simulink model "FirmwareArchitecture"  (R2024a)
settings: Solver=FixedStepDiscrete  StartTime=0.0  StopTime=10.0  RelTol=1e-3
settings Model: DataDictionary=data_definitions.sldd  Creator=pedro  LastModifiedBy=pedro

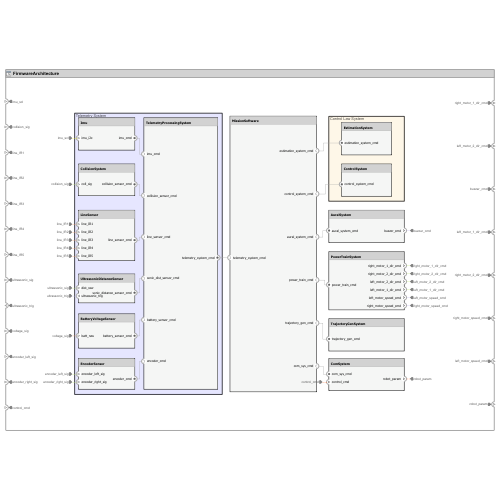
[thumbnail: Simulink's stored preview of the top-level diagram]
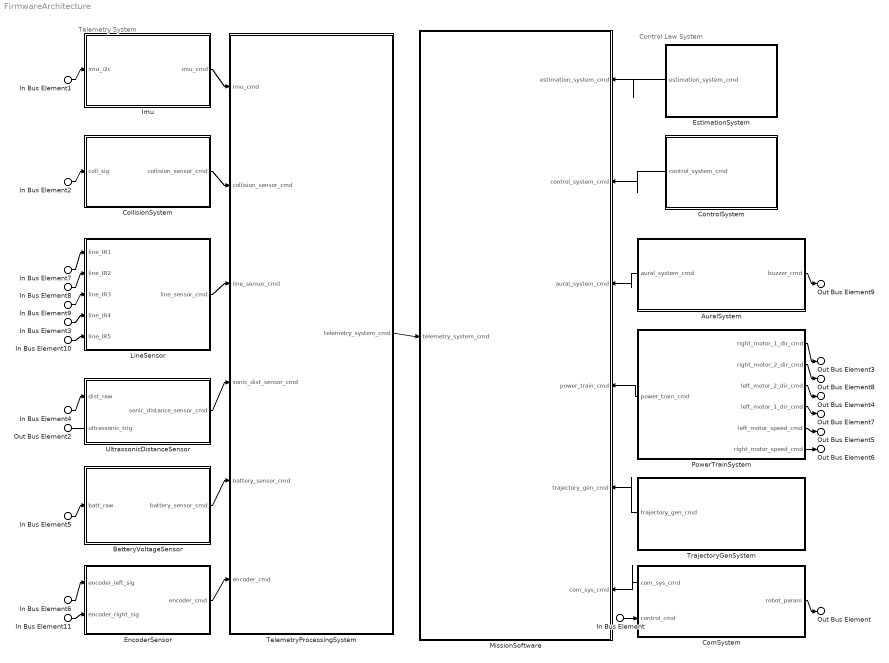
== system FirmwareArchitecture ==
  note: Control Law System
  note: Telemetry System
  In Bus Element1 : Inport  PortName=imu_scl
  In Bus Element2 : Inport  Port=2  PortName=collision_sig
  In Bus Element7 : Inport  Port=3  PortName=line_IR1
  In Bus Element8 : Inport  Port=4  PortName=line_IR2
  In Bus Element9 : Inport  Port=5  PortName=line_IR3
  In Bus Element3 : Inport  Port=6  PortName=line_IR4
  In Bus Element10 : Inport  Port=7  PortName=line_IR5
  In Bus Element4 : Inport  Port=8  PortName=ultrassonic_sig
  In Bus Element5 : Inport  Port=9  PortName=voltage_sig
  In Bus Element6 : Inport  Port=10  PortName=encoder_left_sig
  In Bus Element11 : Inport  Port=11  PortName=encoder_right_sig
  In Bus Element : Inport  Port=12  PortName=control_cmd
  AuralSystem : Subsystem
      settings: PortSchema="{\"entries\":[{\"content\":{\"headerSize\":26,\"margin\":15,\"minimumSpacing\":25,\"sides\":[{\"content\":{\"connectorIds\":[\"Out2\"]},\"type\":\"ConnectorPlacement.EquallySpacedRectSide\",\"uuid\":\"4d6c5e10-6186-41fb-b2bf-ba98d7aba04e\"},{\"content\":{\"connectorIds\":[\"Out1\"],\"side\":\"RIGHT\"},\"type\":\"ConnectorPlacement.EquallySpacedRectSide\",\"uuid\":\"376cbcb5-ae00-4ee4-b51a-d7e41488d4d0\"},{\"content\":{\"side\":\"TOP\"},\"type\":\"ConnectorPlacement.EquallySpacedRectSide\",\"uuid\":\"7d78b6f2-ded8-4819-b676-701e54dd8720\"}]},\"type\":\"ConnectorPlacement.EquallySpacedConnector\",\"uuid\":\"61036d85-7ed2-4698-95df-f6a26735d595\"}],\"packageUris\":[\"http://schema.mathworks.com/mf0/Connector/R2020b\"],\"version\":\"1.0\"}"
  BatteryVoltageSensor : Subsystem
      settings: PortSchema="{\"entries\":[{\"content\":{\"headerSize\":26,\"margin\":15,\"minimumSpacing\":25,\"sides\":[{\"content\":{\"connectorIds\":[\"In1\"]},\"type\":\"ConnectorPlacement.EquallySpacedRectSide\",\"uuid\":\"4d6c5e10-6186-41fb-b2bf-ba98d7aba04e\"},{\"content\":{\"connectorIds\":[\"Out1\"],\"side\":\"RIGHT\"},\"type\":\"ConnectorPlacement.EquallySpacedRectSide\",\"uuid\":\"376cbcb5-ae00-4ee4-b51a-d7e41488d4d0\"},{\"content\":{\"side\":\"TOP\"},\"type\":\"ConnectorPlacement.EquallySpacedRectSide\",\"uuid\":\"7d78b6f2-ded8-4819-b676-701e54dd8720\"}]},\"type\":\"ConnectorPlacement.EquallySpacedConnector\",\"uuid\":\"61036d85-7ed2-4698-95df-f6a26735d595\"}],\"packageUris\":[\"http://schema.mathworks.com/mf0/Connector/R2020b\"],\"version\":\"1.0\"}"
  CollisionSystem : Subsystem
      settings: PortSchema="{\"entries\":[{\"content\":{\"headerSize\":26,\"margin\":15,\"minimumSpacing\":25,\"sides\":[{\"content\":{\"connectorIds\":[\"In1\"]},\"type\":\"ConnectorPlacement.EquallySpacedRectSide\",\"uuid\":\"4d6c5e10-6186-41fb-b2bf-ba98d7aba04e\"},{\"content\":{\"connectorIds\":[\"Out1\"],\"side\":\"RIGHT\"},\"type\":\"ConnectorPlacement.EquallySpacedRectSide\",\"uuid\":\"376cbcb5-ae00-4ee4-b51a-d7e41488d4d0\"},{\"content\":{\"side\":\"TOP\"},\"type\":\"ConnectorPlacement.EquallySpacedRectSide\",\"uuid\":\"7d78b6f2-ded8-4819-b676-701e54dd8720\"}]},\"type\":\"ConnectorPlacement.EquallySpacedConnector\",\"uuid\":\"61036d85-7ed2-4698-95df-f6a26735d595\"}],\"packageUris\":[\"http://schema.mathworks.com/mf0/Connector/R2020b\"],\"version\":\"1.0\"}"
  ComSystem : Subsystem
      settings: PortSchema="{\"entries\":[{\"content\":{\"headerSize\":26,\"margin\":15,\"minimumSpacing\":25,\"sides\":[{\"content\":{\"connectorIds\":[\"Out2\",\"In1\"]},\"type\":\"ConnectorPlacement.EquallySpacedRectSide\",\"uuid\":\"4d6c5e10-6186-41fb-b2bf-ba98d7aba04e\"},{\"content\":{\"connectorIds\":[\"Out1\"],\"side\":\"RIGHT\"},\"type\":\"ConnectorPlacement.EquallySpacedRectSide\",\"uuid\":\"376cbcb5-ae00-4ee4-b51a-d7e41488d4d0\"},{\"content\":{\"side\":\"TOP\"},\"type\":\"ConnectorPlacement.EquallySpacedRectSide\",\"uuid\":\"7d78b6f2-ded8-4819-b676-701e54dd8720\"}]},\"type\":\"ConnectorPlacement.EquallySpacedConnector\",\"uuid\":\"61036d85-7ed2-4698-95df-f6a26735d595\"}],\"packageUris\":[\"http://schema.mathworks.com/mf0/Connector/R2020b\"],\"version\":\"1.0\"}"
  ControlSystem : Subsystem
      settings: PortSchema="{\"entries\":[{\"content\":{\"headerSize\":26,\"margin\":15,\"minimumSpacing\":25,\"sides\":[{\"content\":{\"connectorIds\":[\"Out1\"]},\"type\":\"ConnectorPlacement.EquallySpacedRectSide\",\"uuid\":\"4d6c5e10-6186-41fb-b2bf-ba98d7aba04e\"},{\"content\":{\"side\":\"RIGHT\"},\"type\":\"ConnectorPlacement.EquallySpacedRectSide\",\"uuid\":\"376cbcb5-ae00-4ee4-b51a-d7e41488d4d0\"},{\"content\":{\"side\":\"TOP\"},\"type\":\"ConnectorPlacement.EquallySpacedRectSide\",\"uuid\":\"7d78b6f2-ded8-4819-b676-701e54dd8720\"}]},\"type\":\"ConnectorPlacement.EquallySpacedConnector\",\"uuid\":\"61036d85-7ed2-4698-95df-f6a26735d595\"}],\"packageUris\":[\"http://schema.mathworks.com/mf0/Connector/R2020b\"],\"version\":\"1.0\"}"
  EncoderSensor : Subsystem
      settings: PortSchema="{\"entries\":[{\"content\":{\"headerSize\":26,\"margin\":15,\"minimumSpacing\":25,\"sides\":[{\"content\":{\"connectorIds\":[\"In1\",\"In2\"]},\"type\":\"ConnectorPlacement.EquallySpacedRectSide\",\"uuid\":\"4d6c5e10-6186-41fb-b2bf-ba98d7aba04e\"},{\"content\":{\"connectorIds\":[\"Out1\"],\"side\":\"RIGHT\"},\"type\":\"ConnectorPlacement.EquallySpacedRectSide\",\"uuid\":\"376cbcb5-ae00-4ee4-b51a-d7e41488d4d0\"},{\"content\":{\"side\":\"TOP\"},\"type\":\"ConnectorPlacement.EquallySpacedRectSide\",\"uuid\":\"7d78b6f2-ded8-4819-b676-701e54dd8720\"}]},\"type\":\"ConnectorPlacement.EquallySpacedConnector\",\"uuid\":\"61036d85-7ed2-4698-95df-f6a26735d595\"}],\"packageUris\":[\"http://schema.mathworks.com/mf0/Connector/R2020b\"],\"version\":\"1.0\"}"
  EstimationSystem : Subsystem
      settings: PortSchema="{\"entries\":[{\"content\":{\"headerSize\":26,\"margin\":15,\"minimumSpacing\":25,\"sides\":[{\"content\":{\"connectorIds\":[\"Out1\"]},\"type\":\"ConnectorPlacement.EquallySpacedRectSide\",\"uuid\":\"4d6c5e10-6186-41fb-b2bf-ba98d7aba04e\"},{\"content\":{\"side\":\"RIGHT\"},\"type\":\"ConnectorPlacement.EquallySpacedRectSide\",\"uuid\":\"376cbcb5-ae00-4ee4-b51a-d7e41488d4d0\"},{\"content\":{\"side\":\"TOP\"},\"type\":\"ConnectorPlacement.EquallySpacedRectSide\",\"uuid\":\"7d78b6f2-ded8-4819-b676-701e54dd8720\"}]},\"type\":\"ConnectorPlacement.EquallySpacedConnector\",\"uuid\":\"61036d85-7ed2-4698-95df-f6a26735d595\"}],\"packageUris\":[\"http://schema.mathworks.com/mf0/Connector/R2020b\"],\"version\":\"1.0\"}"
  Imu : Subsystem
      settings: PortSchema="{\"entries\":[{\"content\":{\"headerSize\":26,\"margin\":15,\"minimumSpacing\":25,\"sides\":[{\"content\":{\"connectorIds\":[\"In1\"]},\"type\":\"ConnectorPlacement.EquallySpacedRectSide\",\"uuid\":\"4d6c5e10-6186-41fb-b2bf-ba98d7aba04e\"},{\"content\":{\"connectorIds\":[\"Out1\"],\"side\":\"RIGHT\"},\"type\":\"ConnectorPlacement.EquallySpacedRectSide\",\"uuid\":\"376cbcb5-ae00-4ee4-b51a-d7e41488d4d0\"},{\"content\":{\"side\":\"TOP\"},\"type\":\"ConnectorPlacement.EquallySpacedRectSide\",\"uuid\":\"7d78b6f2-ded8-4819-b676-701e54dd8720\"}]},\"type\":\"ConnectorPlacement.EquallySpacedConnector\",\"uuid\":\"61036d85-7ed2-4698-95df-f6a26735d595\"}],\"packageUris\":[\"http://schema.mathworks.com/mf0/Connector/R2020b\"],\"version\":\"1.0\"}"
  LineSensor : Subsystem
      settings: PortSchema="{\"entries\":[{\"content\":{\"headerSize\":26,\"margin\":15,\"minimumSpacing\":25,\"sides\":[{\"content\":{\"connectorIds\":[\"In1\",\"In2\",\"In3\",\"In4\",\"In5\"]},\"type\":\"ConnectorPlacement.EquallySpacedRectSide\",\"uuid\":\"4d6c5e10-6186-41fb-b2bf-ba98d7aba04e\"},{\"content\":{\"connectorIds\":[\"Out1\"],\"side\":\"RIGHT\"},\"type\":\"ConnectorPlacement.EquallySpacedRectSide\",\"uuid\":\"376cbcb5-ae00-4ee4-b51a-d7e41488d4d0\"},{\"content\":{\"side\":\"TOP\"},\"type\":\"ConnectorPlacement.EquallySpacedRectSide\",\"uuid\":\"7d78b6f2-ded8-4819-b676-701e54dd8720\"}]},\"type\":\"ConnectorPlacement.EquallySpacedConnector\",\"uuid\":\"61036d85-7ed2-4698-95df-f6a26735d595\"}],\"packageUris\":[\"http://schema.mathworks.com/mf0/Connector/R2020b\"],\"version\":\"1.0\"}"
  MissionSoftware : Subsystem
      settings: PortSchema="{\"entries\":[{\"content\":{\"headerSize\":26,\"margin\":15,\"minimumSpacing\":25,\"sides\":[{\"content\":{\"connectorIds\":[\"In6\"]},\"type\":\"ConnectorPlacement.EquallySpacedRectSide\",\"uuid\":\"4d6c5e10-6186-41fb-b2bf-ba98d7aba04e\"},{\"content\":{\"connectorIds\":[\"In1\",\"In2\",\"In3\",\"In4\",\"In5\",\"In7\"],\"side\":\"RIGHT\"},\"type\":\"ConnectorPlacement.EquallySpacedRectSide\",\"uuid\":\"376cbcb5-ae00-4ee4-b51a-d7e41488d4d0\"},{\"content\":{\"side\":\"TOP\"},\"type\":\"ConnectorPlacement.EquallySpacedRectSide\",\"uuid\":\"7d78b6f2-ded8-4819-b676-701e54dd8720\"}]},\"type\":\"ConnectorPlacement.EquallySpacedConnector\",\"uuid\":\"61036d85-7ed2-4698-95df-f6a26735d595\"}],\"packageUris\":[\"http://schema.mathworks.com/mf0/Connector/R2020b\"],\"version\":\"1.0\"}"
  PowerTrainSystem : Subsystem
      settings: PortSchema="{\"entries\":[{\"content\":{\"headerSize\":26,\"margin\":15,\"minimumSpacing\":25,\"sides\":[{\"content\":{\"connectorIds\":[\"Out7\"]},\"type\":\"ConnectorPlacement.EquallySpacedRectSide\",\"uuid\":\"4d6c5e10-6186-41fb-b2bf-ba98d7aba04e\"},{\"content\":{\"connectorIds\":[\"Out1\",\"Out4\",\"Out2\",\"Out3\",\"Out6\",\"Out5\"],\"side\":\"RIGHT\"},\"type\":\"ConnectorPlacement.EquallySpacedRectSide\",\"uuid\":\"376cbcb5-ae00-4ee4-b51a-d7e41488d4d0\"},{\"content\":{\"side\":\"TOP\"},\"type\":\"ConnectorPlacement.EquallySpacedRectSide\",\"uuid\":\"7d78b6f2-ded8-4819-b676-701e54dd8720\"}]},\"type\":\"ConnectorPlacement.EquallySpacedConnector\",\"uuid\":\"61036d85-7ed2-4698-95df-f6a26735d595\"}],\"packageUris\":[\"http://schema.mathworks.com/mf0/Connector/R2020b\"],\"version\":\"1.0\"}"
  TelemetryProcessingSystem : Subsystem
      settings: PortSchema="{\"entries\":[{\"content\":{\"headerSize\":26,\"margin\":15,\"minimumSpacing\":25,\"sides\":[{\"content\":{\"connectorIds\":[\"In1\",\"In3\",\"In2\",\"In4\",\"In5\",\"In6\"]},\"type\":\"ConnectorPlacement.EquallySpacedRectSide\",\"uuid\":\"4d6c5e10-6186-41fb-b2bf-ba98d7aba04e\"},{\"content\":{\"connectorIds\":[\"Out1\"],\"side\":\"RIGHT\"},\"type\":\"ConnectorPlacement.EquallySpacedRectSide\",\"uuid\":\"376cbcb5-ae00-4ee4-b51a-d7e41488d4d0\"},{\"content\":{\"side\":\"TOP\"},\"type\":\"ConnectorPlacement.EquallySpacedRectSide\",\"uuid\":\"7d78b6f2-ded8-4819-b676-701e54dd8720\"}]},\"type\":\"ConnectorPlacement.EquallySpacedConnector\",\"uuid\":\"61036d85-7ed2-4698-95df-f6a26735d595\"}],\"packageUris\":[\"http://schema.mathworks.com/mf0/Connector/R2020b\"],\"version\":\"1.0\"}"
  TrajectoryGenSystem : Subsystem
      settings: PortSchema="{\"entries\":[{\"content\":{\"headerSize\":26,\"margin\":15,\"minimumSpacing\":25,\"sides\":[{\"content\":{\"connectorIds\":[\"Out1\"]},\"type\":\"ConnectorPlacement.EquallySpacedRectSide\",\"uuid\":\"4d6c5e10-6186-41fb-b2bf-ba98d7aba04e\"},{\"content\":{\"side\":\"RIGHT\"},\"type\":\"ConnectorPlacement.EquallySpacedRectSide\",\"uuid\":\"376cbcb5-ae00-4ee4-b51a-d7e41488d4d0\"},{\"content\":{\"side\":\"TOP\"},\"type\":\"ConnectorPlacement.EquallySpacedRectSide\",\"uuid\":\"7d78b6f2-ded8-4819-b676-701e54dd8720\"}]},\"type\":\"ConnectorPlacement.EquallySpacedConnector\",\"uuid\":\"61036d85-7ed2-4698-95df-f6a26735d595\"}],\"packageUris\":[\"http://schema.mathworks.com/mf0/Connector/R2020b\"],\"version\":\"1.0\"}"
  UltrassonicDistanceSensor : Subsystem
      settings: PortSchema="{\"entries\":[{\"content\":{\"headerSize\":26,\"margin\":15,\"minimumSpacing\":25,\"sides\":[{\"content\":{\"connectorIds\":[\"In1\",\"Out2\"]},\"type\":\"ConnectorPlacement.EquallySpacedRectSide\",\"uuid\":\"4d6c5e10-6186-41fb-b2bf-ba98d7aba04e\"},{\"content\":{\"connectorIds\":[\"Out1\"],\"side\":\"RIGHT\"},\"type\":\"ConnectorPlacement.EquallySpacedRectSide\",\"uuid\":\"376cbcb5-ae00-4ee4-b51a-d7e41488d4d0\"},{\"content\":{\"side\":\"TOP\"},\"type\":\"ConnectorPlacement.EquallySpacedRectSide\",\"uuid\":\"7d78b6f2-ded8-4819-b676-701e54dd8720\"}]},\"type\":\"ConnectorPlacement.EquallySpacedConnector\",\"uuid\":\"61036d85-7ed2-4698-95df-f6a26735d595\"}],\"packageUris\":[\"http://schema.mathworks.com/mf0/Connector/R2020b\"],\"version\":\"1.0\"}"
  Out Bus Element3 : Outport  PortName=right_motor_1_dir_cmd
  Out Bus Element4 : Outport  Port=2  PortName=left_motor_2_dir_cmd
  Out Bus Element9 : Outport  Port=3  PortName=buzzer_cmd
  Out Bus Element7 : Outport  Port=4  PortName=left_motor_1_dir_cmd
  Out Bus Element8 : Outport  Port=5  PortName=right_motor_2_dir_cmd
  Out Bus Element6 : Outport  Port=6  PortName=right_motor_speed_cmd
  Out Bus Element5 : Outport  Port=7  PortName=left_motor_speed_cmd
  Out Bus Element2 : Outport  Port=8  PortName=ultrassonic_trig
  Out Bus Element : Outport  Port=9  PortName=robot_param
  wires:
  Imu/1(imu_cmd) -> TelemetryProcessingSystem/1(imu_cmd)
  CollisionSystem/1(collision_sensor_cmd) -> TelemetryProcessingSystem/3(collision_sensor_cmd)
  LineSensor/1(line_sensor_cmd) -> TelemetryProcessingSystem/2(line_sensor_cmd)
  UltrassonicDistanceSensor/1(sonic_distance_sensor_cmd) -> TelemetryProcessingSystem/4(sonic_dist_sensor_cmd)
  BatteryVoltageSensor/1(battery_sensor_cmd) -> TelemetryProcessingSystem/5(battery_sensor_cmd)
  EncoderSensor/1(encoder_cmd) -> TelemetryProcessingSystem/6(encoder_cmd)
  ComSystem/2(com_sys_cmd) -> MissionSoftware/7(com_sys_cmd)
  TelemetryProcessingSystem/1(telemetry_system_cmd) -> MissionSoftware/6(telemetry_system_cmd)
  EstimationSystem/1(estimation_system_cmd) -> MissionSoftware/1(estimation_system_cmd)
  ControlSystem/1(control_system_cmd) -> MissionSoftware/2(control_system_cmd)
  TrajectoryGenSystem/1(trajectory_gen_cmd) -> MissionSoftware/5(trajectory_gen_cmd)
  ComSystem/1(robot_param) -> Out Bus Element/1
  In Bus Element/1 -> ComSystem/1(control_cmd)
  In Bus Element1/1 -> Imu/1(imu_i2c)
  In Bus Element2/1 -> CollisionSystem/1(coll_sig)
  In Bus Element3/1 -> LineSensor/4(line_IR4)
  In Bus Element4/1 -> UltrassonicDistanceSensor/1(dist_raw)
  In Bus Element5/1 -> BatteryVoltageSensor/1(batt_raw)
  In Bus Element6/1 -> EncoderSensor/1(encoder_left_sig)
  In Bus Element7/1 -> LineSensor/1(line_IR1)
  In Bus Element8/1 -> LineSensor/2(line_IR2)
  In Bus Element9/1 -> LineSensor/3(line_IR3)
  In Bus Element10/1 -> LineSensor/5(line_IR5)
  UltrassonicDistanceSensor/2(ultrassonic_trig) -> Out Bus Element2/1
  In Bus Element11/1 -> EncoderSensor/2(encoder_right_sig)
  PowerTrainSystem/1(right_motor_1_dir_cmd) -> Out Bus Element3/1
  PowerTrainSystem/2(left_motor_2_dir_cmd) -> Out Bus Element4/1
  PowerTrainSystem/6(left_motor_speed_cmd) -> Out Bus Element5/1
  PowerTrainSystem/5(right_motor_speed_cmd) -> Out Bus Element6/1
  PowerTrainSystem/7(power_train_cmd) -> MissionSoftware/4(power_train_cmd)
  PowerTrainSystem/3(left_motor_1_dir_cmd) -> Out Bus Element7/1
  PowerTrainSystem/4(right_motor_2_dir_cmd) -> Out Bus Element8/1
  AuralSystem/2(aural_system_cmd) -> MissionSoftware/3(aural_system_cmd)
  AuralSystem/1(buzzer_cmd) -> Out Bus Element9/1

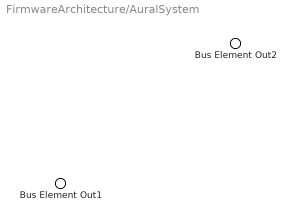
== system FirmwareArchitecture/AuralSystem ==
  Bus Element Out2 : Outport  PortName=buzzer_cmd
  Bus Element Out1 : Outport  Port=2  AllowServiceAccess=on  PortName=aural_system_cmd

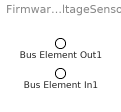
== system FirmwareArchitecture/BatteryVoltageSensor ==
  Bus Element In1 : Inport  PortName=batt_raw
  Bus Element Out1 : Outport  AllowServiceAccess=on  PortName=battery_sensor_cmd

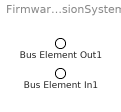
== system FirmwareArchitecture/CollisionSystem ==
  Bus Element In1 : Inport  PortName=coll_sig
  Bus Element Out1 : Outport  AllowServiceAccess=on  PortName=collision_sensor_cmd

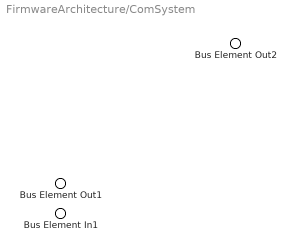
== system FirmwareArchitecture/ComSystem ==
  Bus Element In1 : Inport  PortName=control_cmd
  Bus Element Out2 : Outport  PortName=robot_param
  Bus Element Out1 : Outport  Port=2  AllowServiceAccess=on  PortName=com_sys_cmd

== system FirmwareArchitecture/ControlSystem ==
  Bus Element Out1 : Outport  AllowServiceAccess=on  PortName=control_system_cmd

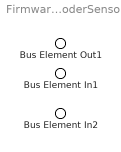
== system FirmwareArchitecture/EncoderSensor ==
  Bus Element In1 : Inport  PortName=encoder_left_sig
  Bus Element In2 : Inport  Port=2  PortName=encoder_right_sig
  Bus Element Out1 : Outport  AllowServiceAccess=on  PortName=encoder_cmd

== system FirmwareArchitecture/EstimationSystem ==
  Bus Element Out1 : Outport  AllowServiceAccess=on  PortName=estimation_system_cmd

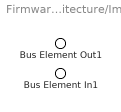
== system FirmwareArchitecture/Imu ==
  Bus Element In1 : Inport  PortName=imu_i2c
  Bus Element Out1 : Outport  AllowServiceAccess=on  PortName=imu_cmd

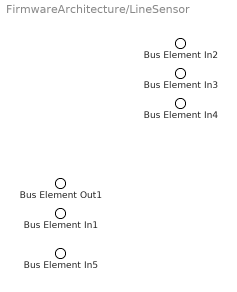
== system FirmwareArchitecture/LineSensor ==
  Bus Element In2 : Inport  PortName=line_IR1
  Bus Element In3 : Inport  Port=2  PortName=line_IR2
  Bus Element In4 : Inport  Port=3  PortName=line_IR3
  Bus Element In1 : Inport  Port=4  PortName=line_IR4
  Bus Element In5 : Inport  Port=5  PortName=line_IR5
  Bus Element Out1 : Outport  AllowServiceAccess=on  PortName=line_sensor_cmd

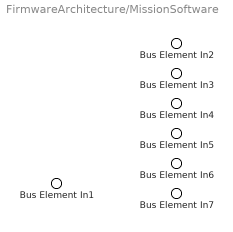
== system FirmwareArchitecture/MissionSoftware ==
  Bus Element In3 : Inport  AllowServiceAccess=on  PortName=estimation_system_cmd
  Bus Element In4 : Inport  Port=2  AllowServiceAccess=on  PortName=control_system_cmd
  Bus Element In7 : Inport  Port=3  AllowServiceAccess=on  PortName=aural_system_cmd
  Bus Element In6 : Inport  Port=4  AllowServiceAccess=on  PortName=power_train_cmd
  Bus Element In5 : Inport  Port=5  AllowServiceAccess=on  PortName=trajectory_gen_cmd
  Bus Element In2 : Inport  Port=6  AllowServiceAccess=on  PortName=telemetry_system_cmd
  Bus Element In1 : Inport  Port=7  AllowServiceAccess=on  PortName=com_sys_cmd

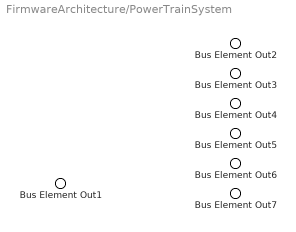
== system FirmwareArchitecture/PowerTrainSystem ==
  Bus Element Out2 : Outport  PortName=right_motor_1_dir_cmd
  Bus Element Out3 : Outport  Port=2  PortName=left_motor_2_dir_cmd
  Bus Element Out6 : Outport  Port=3  PortName=left_motor_1_dir_cmd
  Bus Element Out7 : Outport  Port=4  PortName=right_motor_2_dir_cmd
  Bus Element Out5 : Outport  Port=5  PortName=right_motor_speed_cmd
  Bus Element Out4 : Outport  Port=6  PortName=left_motor_speed_cmd
  Bus Element Out1 : Outport  Port=7  AllowServiceAccess=on  PortName=power_train_cmd

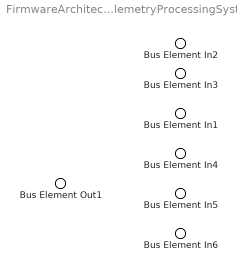
== system FirmwareArchitecture/TelemetryProcessingSystem ==
  Bus Element In2 : Inport  AllowServiceAccess=on  PortName=imu_cmd
  Bus Element In3 : Inport  Port=2  AllowServiceAccess=on  PortName=line_sensor_cmd
  Bus Element In1 : Inport  Port=3  AllowServiceAccess=on  PortName=collision_sensor_cmd
  Bus Element In4 : Inport  Port=4  AllowServiceAccess=on  PortName=sonic_dist_sensor_cmd
  Bus Element In5 : Inport  Port=5  AllowServiceAccess=on  PortName=battery_sensor_cmd
  Bus Element In6 : Inport  Port=6  AllowServiceAccess=on  PortName=encoder_cmd
  Bus Element Out1 : Outport  AllowServiceAccess=on  PortName=telemetry_system_cmd

== system FirmwareArchitecture/TrajectoryGenSystem ==
  Bus Element Out1 : Outport  AllowServiceAccess=on  PortName=trajectory_gen_cmd

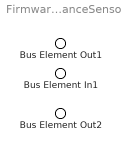
== system FirmwareArchitecture/UltrassonicDistanceSensor ==
  Bus Element In1 : Inport  PortName=dist_raw
  Bus Element Out1 : Outport  AllowServiceAccess=on  PortName=sonic_distance_sensor_cmd
  Bus Element Out2 : Outport  Port=2  PortName=ultrassonic_trig
